simulink model "ESO_test"  (R2013b)
settings: Solver=ode45  StartTime=0.0  StopTime=Tsim  RelTol=1e-3
values from neighbouring files (symbols this model uses):
  A = [-8.94033098083 -936.220139529 0 0 0 0 0 0 936.220139529 -8.94033098083 0 0 ... (64 elements, 8x8)]    [La.mat]    (also in identified_n_8.mat)
  B = B(:,1:2)    [ESO_design_Quadratic_Stabilization.m]    (also in ESO_performance_test.m; La.mat = [3.35350860045 -3.97919586281 -1.08438089314 -3.49556227412 ; identified_n_8.mat = [3.35350860045 -3.97919586281 -1.08438089314 -3.49556227412 )
  C = [0.10097273376 -0.023700638379 0.168405211443 0.241400270211 -0.0208077337143 0.13383372604 0.006626245158 -0.211650251582 -0.022735872456 -0.00189193031132 -0.0174657382815 -0.0972100740962 ... (24 elements, 3x8)]    [La.mat]    (also in identified_n_8.mat)
  D = D(:,1:2)    [ESO_design_Quadratic_Stabilization.m]    (also in ESO_performance_test.m; La.mat = [0.00331165800503  -0.00583155851158; -0.00106885317556  -0.; identified_n_8.mat = [0.00331165800503  -0.00583155851158  -0.00405216167143  -0.)
  E = zeros(nw,nv)    [ESO_design_Quadratic_Stabilization.m]    (also in ESO_performance_test.m; La.mat = [1 1 1 1 1 1 1 1 1 1 1 1])
  F = eye(nv)    [ESO_design_Quadratic_Stabilization.m]    (also in ESO_performance_test.m; La.mat = [1 0 0 0 0 0 0 0 0 0 0 0 ... (144 elements, 12x12)])
  H = B(:,4)    [ESO_design_Quadratic_Stabilization.m]    (also in ESO_performance_test.m; La.mat = [-1.22306207999 1.42132010289 -0.177899777346 2.52414001877 )
  L1 = La(1:nx,:)    [ESO_performance_test.m]
  L2 = La(nx+1:nx+nv,:)    [ESO_performance_test.m]
  nv = size(S,1)    [ESO_design_Quadratic_Stabilization.m]    (also in ESO_performance_test.m; La.mat = 12)
  nx = size(A,1)    [ESO_design_Quadratic_Stabilization.m]    (also in ESO_performance_test.m; La.mat = 8)
  S = [-6.75669916218 -2602.57875791 0 0 0 0 0 0 0 0 0 0 ... (144 elements, 12x12)]    [La.mat]    (also in S.mat)
libraries: simulink x1
settings Model: Creator=Mehran  LastModifiedBy=admin
settings DataIOCC: SignalLoggingSaveFormat=ModelDataLogs
settings OptimizationCC: ExpressionDepthLimit=2147483647
settings DebuggingCC: FcnCallInpInsideContextMsg=UseLocalSettings  StateNameClashWarn=warning
settings GRTTargetCC: CombineOutputUpdateFcns=off  GRTInterface=on

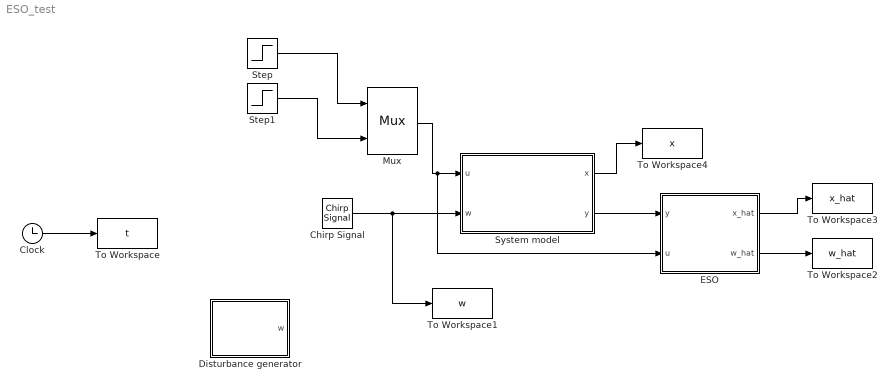
== system ESO_test ==
  Chirp Signal : simulink/Sources/Chirp Signal  f1=0  T=10  f2=100
  Clock : Clock
  Disturbance generator : Subsystem
  ESO : Subsystem
  Mux : Mux  Inputs=2
  Step : Step  Time=0  After=0  SampleTime=0
  Step1 : Step  Time=0  After=0  SampleTime=0
  System model : Subsystem
  To Workspace : ToWorkspace  VariableName=t  SampleTime=-1
  To Workspace1 : ToWorkspace  VariableName=w  SampleTime=-1
  To Workspace2 : ToWorkspace  VariableName=w_hat  SampleTime=-1
  To Workspace3 : ToWorkspace  VariableName=x_hat  SampleTime=-1
  To Workspace4 : ToWorkspace  VariableName=x  SampleTime=-1
  wires:
  System model/2(y) -> ESO/1(y)
  Mux/1 -> System model/1(u), ESO/2(u)
  Step/1 -> Mux/1
  Step1/1 -> Mux/2
  Clock/1 -> To Workspace/1
  ESO/2(w_hat) -> To Workspace2/1
  Chirp Signal/1 -> System model/2(w), To Workspace1/1
  ESO/1(x_hat) -> To Workspace3/1
  System model/1(x) -> To Workspace4/1

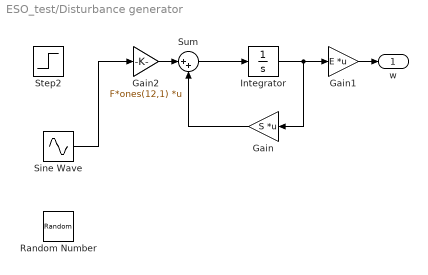
== system ESO_test/Disturbance generator ==
  Gain : Gain  Gain=S  Multiplication=Matrix(K*u)
  Gain1 : Gain  Gain=E  Multiplication=Matrix(K*u)
  Gain2 : Gain  Gain=F*ones(12,1)  Multiplication=Matrix(K*u)
  Integrator : Integrator  InitialCondition=0.1*ones(12,1)
  Random Number : RandomNumber  SampleTime=0.1
  Sine Wave : Sin  Amplitude=3  Frequency=5  SampleTime=0
  Step2 : Step  Time=0  After=0  SampleTime=0
  Sum : Sum  Inputs=|++
  w : Outport
  wires:
  Integrator/1 -> Gain/1, Gain1/1
  Gain/1 -> Sum/2
  Sum/1 -> Integrator/1
  Gain1/1 -> w/1
  Gain2/1 -> Sum/1
  Sine Wave/1 -> Gain2/1

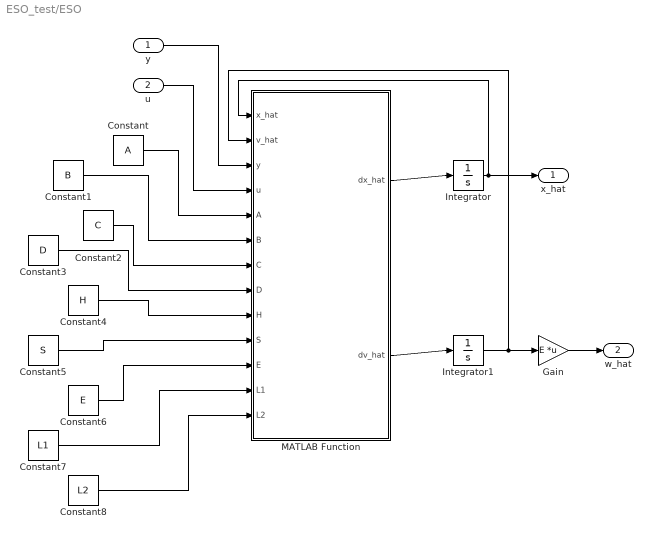
== system ESO_test/ESO ==
  y : Inport
  u : Inport  Port=2
  Constant : Constant  Value=A
  Constant1 : Constant  Value=B
  Constant2 : Constant  Value=C
  Constant3 : Constant  Value=D
  Constant4 : Constant  Value=H
  Constant5 : Constant  Value=S
  Constant6 : Constant  Value=E
  Constant7 : Constant  Value=L1
  Constant8 : Constant  Value=L2
  Gain : Gain  Gain=E  Multiplication=Matrix(K*u)
  Integrator : Integrator  InitialCondition=zeros(nx,1)
  Integrator1 : Integrator  InitialCondition=zeros(nv,1)
  MATLAB Function : MATLAB Function  TreatAsAtomicUnit=on
  x_hat : Outport
  w_hat : Outport  Port=2
  wires:
  MATLAB Function/1(dx_hat) -> Integrator/1
  MATLAB Function/2(dv_hat) -> Integrator1/1
  Integrator/1 -> MATLAB Function/1(x_hat), x_hat/1
  Integrator1/1 -> MATLAB Function/2(v_hat), Gain/1
  y/1 -> MATLAB Function/3(y)
  u/1 -> MATLAB Function/4(u)
  Constant/1 -> MATLAB Function/5(A)
  Constant1/1 -> MATLAB Function/6(B)
  Constant2/1 -> MATLAB Function/7(C)
  Constant3/1 -> MATLAB Function/8(D)
  Constant4/1 -> MATLAB Function/9(H)
  Constant5/1 -> MATLAB Function/10(S)
  Constant6/1 -> MATLAB Function/11(E)
  Constant7/1 -> MATLAB Function/12(L1)
  Constant8/1 -> MATLAB Function/13(L2)
  Gain/1 -> w_hat/1

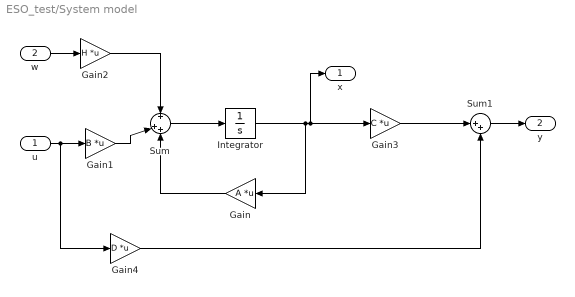
== system ESO_test/System model ==
  u : Inport
  w : Inport  Port=2
  Gain : Gain  Gain=A  Multiplication=Matrix(K*u)
  Gain1 : Gain  Gain=B  Multiplication=Matrix(K*u)
  Gain2 : Gain  Gain=H  Multiplication=Matrix(K*u)
  Gain3 : Gain  Gain=C  Multiplication=Matrix(K*u)
  Gain4 : Gain  Gain=D  Multiplication=Matrix(K*u)
  Integrator : Integrator
  Sum : Sum  Inputs=+|++
  Sum1 : Sum  Inputs=|++
  x : Outport
  y : Outport  Port=2
  wires:
  Sum/1 -> Integrator/1
  Integrator/1 -> Gain3/1, x/1, Gain/1
  Gain/1 -> Sum/3
  Gain1/1 -> Sum/2
  u/1 -> Gain1/1, Gain4/1
  w/1 -> Gain2/1
  Gain2/1 -> Sum/1
  Gain3/1 -> Sum1/1
  Gain4/1 -> Sum1/2
  Sum1/1 -> y/1

== matlab function ESO_test/ESO/MATLAB Function ==
  data: x_hat input; v_hat input; y input; u input; dx_hat output; dv_hat output; A input; B input; C input; D input; H input; S input; E input; L1 input; L2 input
function [dx_hat,dv_hat] = ESO_dyn(x_hat,v_hat,y,u,A,B,C,D,H,S,E,L1,L2)
dx_hat = zeros(8,1);
dv_hat = zeros(12,1);
%% Gain function parameters
a = 0.8;
d = 0.1;
%% ESO DEs
dx_hat = A*x_hat+B*u+(H*E')*v_hat+L1*phi(y-C*x_hat-D*u,a,d);
dv_hat = S*v_hat+L2*phi(y-C*x_hat-D*u,a,d);
end
%Gain function
function y1 = phi(x1,a,d)
         y1 = zeros(3,1);
         y1(1) = x1(1) + 0.5*(a-1)*(abs(x1(1)+d)-abs(x1(1)-d));
         y1(2) = x1(2) + 0.5*(a-1)*(abs(x1(2)+d)-abs(x1(2)-d));
         y1(3) = x1(3) + 0.5*(a-1)*(abs(x1(3)+d)-abs(x1(3)-d));
end
